simulink model "EKF_SIL_02"  (R2015a)
settings: Solver=ode45  StartTime=0.0  StopTime=totalSimulationTime  RelTol=1e-3
model workspace: external: MATLAB File Init_Model_02_Simulink.m (data not in the file)
undefined symbols (not defined in the file): Cov_nu, Cov_r, e_force_x, e_force_y, e_force_z, ieps, ita, lenLinks, n, P_d, P_k, p_x, p_y, p_z, parameter_gravitation, rho, rho_c, sig_f, sig_tau, t_delta, t_Kalman, tau_1, tau_2, tau_3, U_n_d, W_0, X_a_0, x_d, x_k
libraries: simulink x9, aerolibtransform2 x3, dspmtrx3 x2, visionstatistics x1, aerolibutil x1, visionsinks x1
(part 2 of 5)

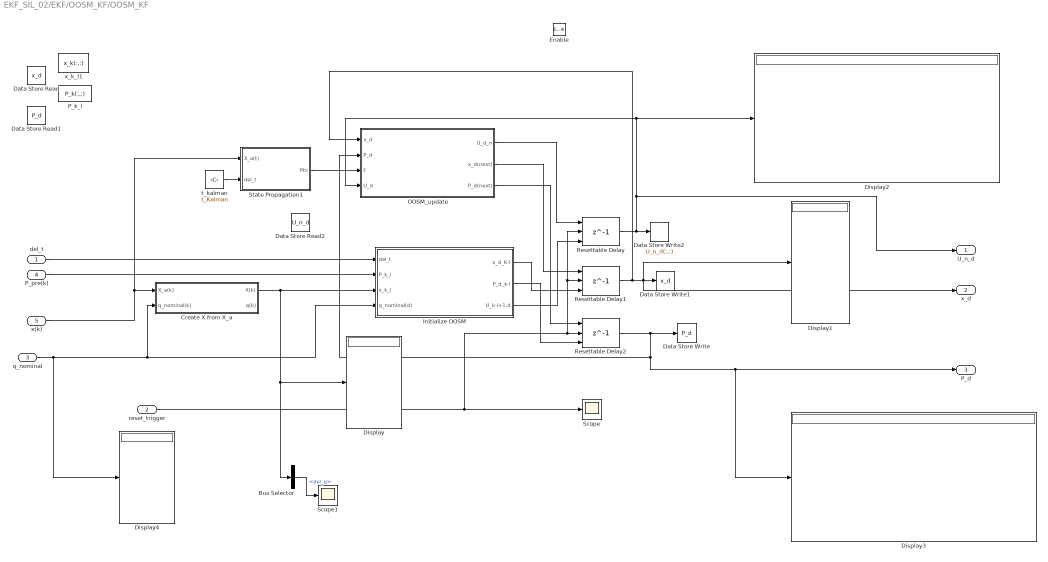
== system EKF_SIL_02/EKF/OOSM_KF/OOSM_KF ==
  del_t : Inport
  reset_trigger : Inport  Port=2
  q_nominal : Inport  Port=3
  P_pre(k) : Inport  Port=4
  "x(k) " : Inport  Port=5
  Enable : EnablePort
  Bus Selector : BusSelector  OutputSignals=del_q
  Create X from X_a : Subsystem
  Data Store Read : DataStoreRead  DataStoreName=x_d
  Data Store Read1 : DataStoreRead  DataStoreName=P_d
  Data Store Read2 : DataStoreRead  DataStoreName=U_n_d
  Data Store Write : DataStoreWrite  DataStoreName=P_d
  Data Store Write1 : DataStoreWrite  DataStoreName=x_d
  Data Store Write2 : DataStoreWrite  DataStoreName=U_n_d  DataStoreElements=U_n_d(:,:)
  Display{,1..4} (5 alike) : Display
  Initialize OOSM : Subsystem  TreatAsAtomicUnit=on
  OOSM_update : Subsystem
  P_k_l : DataStoreRead  DataStoreName=P_k  DataStoreElements=P_k(:,:)
  Resettable Delay : Delay  DelayLength=1  InitialConditionSource=Input port  ExternalReset=Rising
      settings: InputPortMap=u0,r5,p4
  Resettable Delay1 : Delay  DelayLength=1  InitialConditionSource=Input port  ExternalReset=Rising
      settings: InputPortMap=u0,r5,p4
  Resettable Delay2 : Delay  DelayLength=1  InitialConditionSource=Input port  ExternalReset=Rising
      settings: InputPortMap=u0,r5,p4
  Scope : Scope
      settings: SaveName=ScopeData10
  Scope1 : Scope
      settings: YMin=-0.8  YMax=0.4  SaveName=ScopeData17
  State Propagation1 : Subsystem
  t_kalman : Constant  Value=t_Kalman
  x_k_l1 : DataStoreRead  DataStoreName=x_k  DataStoreElements=x_k(:,:)
  U_n_d : Outport
  x_d : Outport  Port=2
  P_d : Outport  Port=3
  wires:
  del_t/1 -> Initialize OOSM/1(del_t)
  Initialize OOSM/3(U_k-l+1,d) -> Resettable Delay/3
  OOSM_update/1(U_d_n) -> Resettable Delay/1
  State Propagation1/1(Phi) -> OOSM_update/3(F)
  t_kalman/1 -> State Propagation1/2(del_t)
  Initialize OOSM/1(x_d_K-l) -> Resettable Delay1/3
  Resettable Delay1/1 -> OOSM_update/1(x_d), x_d/1, Display1/1, Data Store Write1/1
  Resettable Delay2/1 -> OOSM_update/2(P_d), Display3/1, P_d/1, Data Store Write/1
  reset_trigger/1 -> Resettable Delay/2, Resettable Delay1/2, Resettable Delay2/2, Scope/1
  Resettable Delay/1 -> Display2/1, OOSM_update/4("U_d "), U_n_d/1, Data Store Write2/1
  P_pre(k)/1 -> Initialize OOSM/2(P_k_l)
  q_nominal/1 -> Display4/1, Initialize OOSM/4(q_nominal(d)), Create X from X_a/2(q_nominal(k))
  OOSM_update/2(x_d(next)) -> Resettable Delay1/1
  OOSM_update/3(P_d(next)) -> Resettable Delay2/1
  Initialize OOSM/2(P_d_k-l) -> Resettable Delay2/3
  "x(k) "/1 -> State Propagation1/1("X_a(t)\t"), Create X from X_a/1(X_a(k))
  Create X from X_a/1(X(k)) -> Bus Selector/1, Display/1, Initialize OOSM/3(x_k_l)
  Bus Selector/1 -> Scope1/1  "<del_q>"

== system EKF_SIL_02/EKF/OOSM_KF/OOSM_enable ==
  "timestamp_cap " : Inport
  meas_packet : Inport  Port=2
  Bus Selector : BusSelector  OutputSignals=timestamp_processed
  Chart : Stateflow chart  TreatAsAtomicUnit=on
  Create nominal q(d) : Subsystem  TreatAsAtomicUnit=on
  Data Store Write : DataStoreWrite  DialogController=Simulink.DDGSource  DataStoreName=q_nominal_d
  Delay : Delay  DelayLength=1  InitialCondition=0
  Delay1 : Delay  DelayLength=1  InitialCondition=0
  Detect Increase : simulink/Logic and Bit Operations/Detect Increase  vinit=-1  InputProcessing=Inherited  OutDataTypeStr=boolean
  Detect Increase1 : simulink/Logic and Bit Operations/Detect Increase  vinit=-1  InputProcessing=Inherited  OutDataTypeStr=boolean
  Display : Display
  Enabled Subsystem : Subsystem  TreatAsAtomicUnit=on
  IC : InitialCondition  Value=-1
  IC1 : InitialCondition  Value=-1
  Mux : Mux  Inputs=2
  Scope : Scope
      settings: SaveName=ScopeData16
  Trigger : Outport
  reset_trigger : Outport  Port=2
  "q_nominal " : Outport  Port=3
  wires:
  Mux/1 -> Chart/Trigger
  Bus Selector/1 -> IC1/1  "<timestamp_processed>"
  meas_packet/1 -> Bus Selector/1
  IC1/1 -> Detect Increase1/1
  Detect Increase/1 -> Create nominal q(d)/Trigger, Delay/1  "camera_cap"
  Chart/1(out) -> Scope/1, Trigger/1
  "timestamp_cap "/1 -> IC/1
  IC/1 -> Create nominal q(d)/1(timestamp_cap), Detect Increase/1
  Detect Increase1/1 -> Delay1/1  "meas_arrived"
  Create nominal q(d)/1(q_nominal) -> Display/1, Data Store Write/1, "q_nominal "/1
  Delay/1 -> Mux/2, reset_trigger/1
  Delay1/1 -> Mux/1

== system EKF_SIL_02/EKF/Predictor/Create Bus [State Vector,X_a] ==
  X : Inport
  Bus Creator2 : BusCreator
  Bus Creator3 : BusCreator  Inputs=3
  Bus Creator4 : BusCreator  Inputs=3
  Bus Creator5 : BusCreator  Inputs=3
  Bus Creator6 : BusCreator
  Demux1 : Demux  Outputs=13
  X_bus : Outport
  wires:
  Bus Creator2/1 -> Bus Creator6/1  "q_est"
  Bus Creator3/1 -> Bus Creator6/2  "omega"
  Bus Creator4/1 -> Bus Creator6/3  "r"
  Bus Creator5/1 -> Bus Creator6/4  "r_dot"
  Bus Creator6/1 -> X_bus/1
  X/1 -> Demux1/1
  Demux1/1 -> Bus Creator2/1  "q_est_1"
  Demux1/2 -> Bus Creator2/2  "q_est_2"
  Demux1/3 -> Bus Creator2/3  "q_est_3"
  Demux1/4 -> Bus Creator2/4  "q_est_0"
  Demux1/5 -> Bus Creator3/1  "omega_x"
  Demux1/6 -> Bus Creator3/2  "omega_y"
  Demux1/7 -> Bus Creator3/3  "omega_z"
  Demux1/8 -> Bus Creator4/1  "r_x"
  Demux1/9 -> Bus Creator4/2  "r_y"
  Demux1/10 -> Bus Creator4/3  "r_z"
  Demux1/11 -> Bus Creator5/1  "r_x_dot"
  Demux1/12 -> Bus Creator5/2  "r_y_dot"
  Demux1/13 -> Bus Creator5/3  "r_z_dot"

== system EKF_SIL_02/EKF/Predictor/Create Bus [State Vector,X_a]1 ==
  X : Inport
  Bus Creator2 : BusCreator
  Bus Creator3 : BusCreator  Inputs=3
  Bus Creator4 : BusCreator  Inputs=3
  Bus Creator5 : BusCreator  Inputs=3
  Bus Creator6 : BusCreator
  Demux1 : Demux  Outputs=13
  X_bus : Outport
  wires:
  Demux1/13 -> Bus Creator5/3  "r_z_dot"
  Demux1/12 -> Bus Creator5/2  "r_y_dot"
  Demux1/11 -> Bus Creator5/1  "r_x_dot"
  Demux1/10 -> Bus Creator4/3  "r_z"
  Demux1/9 -> Bus Creator4/2  "r_y"
  Demux1/8 -> Bus Creator4/1  "r_x"
  Demux1/7 -> Bus Creator3/3  "omega_z"
  Demux1/6 -> Bus Creator3/2  "omega_y"
  Demux1/5 -> Bus Creator3/1  "omega_x"
  Demux1/4 -> Bus Creator2/4  "q_est_0"
  Demux1/3 -> Bus Creator2/3  "q_est_3"
  Demux1/2 -> Bus Creator2/2  "q_est_2"
  Demux1/1 -> Bus Creator2/1  "q_est_1"
  X/1 -> Demux1/1
  Bus Creator6/1 -> X_bus/1
  Bus Creator5/1 -> Bus Creator6/4  "r_dot"
  Bus Creator4/1 -> Bus Creator6/3  "r"
  Bus Creator3/1 -> Bus Creator6/2  "omega"
  Bus Creator2/1 -> Bus Creator6/1  "q_est"

== system EKF_SIL_02/EKF/Predictor/Create Bus [State Vector,X_a]2 ==
  X : Inport
  Bus Creator2 : BusCreator
  Bus Creator3 : BusCreator  Inputs=3
  Bus Creator4 : BusCreator  Inputs=3
  Bus Creator5 : BusCreator  Inputs=3
  Bus Creator6 : BusCreator
  Demux1 : Demux  Outputs=13
  X_bus : Outport
  wires:
  Demux1/13 -> Bus Creator5/3  "r_z_dot"
  Demux1/12 -> Bus Creator5/2  "r_y_dot"
  Demux1/11 -> Bus Creator5/1  "r_x_dot"
  Demux1/10 -> Bus Creator4/3  "r_z"
  Demux1/9 -> Bus Creator4/2  "r_y"
  Demux1/8 -> Bus Creator4/1  "r_x"
  Demux1/7 -> Bus Creator3/3  "omega_z"
  Demux1/6 -> Bus Creator3/2  "omega_y"
  Demux1/5 -> Bus Creator3/1  "omega_x"
  Demux1/4 -> Bus Creator2/4  "q_est_0"
  Demux1/3 -> Bus Creator2/3  "q_est_3"
  Demux1/2 -> Bus Creator2/2  "q_est_2"
  Demux1/1 -> Bus Creator2/1  "q_est_1"
  X/1 -> Demux1/1
  Bus Creator6/1 -> X_bus/1
  Bus Creator5/1 -> Bus Creator6/4  "r_dot"
  Bus Creator4/1 -> Bus Creator6/3  "r"
  Bus Creator3/1 -> Bus Creator6/2  "omega"
  Bus Creator2/1 -> Bus Creator6/1  "q_est"

== system EKF_SIL_02/EKF/Predictor/Create Bus [State Vector,X_a]3 ==
  X : Inport
  Bus Creator2 : BusCreator
  Bus Creator3 : BusCreator  Inputs=3
  Bus Creator4 : BusCreator  Inputs=3
  Bus Creator5 : BusCreator  Inputs=3
  Bus Creator6 : BusCreator
  Demux1 : Demux  Outputs=13
  X_bus : Outport
  wires:
  Bus Creator2/1 -> Bus Creator6/1  "q_est"
  Bus Creator3/1 -> Bus Creator6/2  "omega"
  Bus Creator4/1 -> Bus Creator6/3  "r"
  Bus Creator5/1 -> Bus Creator6/4  "r_dot"
  Bus Creator6/1 -> X_bus/1
  X/1 -> Demux1/1
  Demux1/1 -> Bus Creator2/1  "q_est_1"
  Demux1/2 -> Bus Creator2/2  "q_est_2"
  Demux1/3 -> Bus Creator2/3  "q_est_3"
  Demux1/4 -> Bus Creator2/4  "q_est_0"
  Demux1/5 -> Bus Creator3/1  "omega_x"
  Demux1/6 -> Bus Creator3/2  "omega_y"
  Demux1/7 -> Bus Creator3/3  "omega_z"
  Demux1/8 -> Bus Creator4/1  "r_x"
  Demux1/9 -> Bus Creator4/2  "r_y"
  Demux1/10 -> Bus Creator4/3  "r_z"
  Demux1/11 -> Bus Creator5/1  "r_x_dot"
  Demux1/12 -> Bus Creator5/2  "r_y_dot"
  Demux1/13 -> Bus Creator5/3  "r_z_dot"

== system EKF_SIL_02/EKF/Predictor/Create State error covariance (P) ==
  X_a : Inport
  P_previous : Inport  Port=2
  Add : Sum
  Math Function : Math  Operator=transpose  SaturateOnIntegerOverflow=on
  Matrix Concatenate : Concatenate  Mode=Multidimensional array  ConcatenateDimension=2
  Matrix Concatenate1 : Concatenate  Mode=Multidimensional array
  Matrix Concatenate2 : Concatenate  Mode=Multidimensional array  ConcatenateDimension=2
  Process noise covariance [rotational] : Subsystem
  Process noise covariance [translational] : Subsystem
  Product : Product  Inputs=3  Multiplication=Matrix(*)
  State Propagation : Subsystem
  zeros(6,6) : Constant  Value=zeros(6,6)
  P_current : Outport
  wires:
  Math Function/1 -> Product/3
  P_previous/1 -> Product/2
  Add/1 -> P_current/1
  X_a/1 -> State Propagation/1("X_a(t)\t")
  Product/1 -> Add/2
  Matrix Concatenate1/1 -> Add/1
  Matrix Concatenate2/1 -> Matrix Concatenate1/2
  Matrix Concatenate/1 -> Matrix Concatenate1/1
  Process noise covariance [translational]/1(Q_t) -> Matrix Concatenate2/2
  zeros(6,6)/1 -> Matrix Concatenate2/1, Matrix Concatenate/2
  Process noise covariance [rotational]/1(Q_r) -> Matrix Concatenate/1
  State Propagation/1(Phi) -> Math Function/1, Product/1, Process noise covariance [rotational]/1(Phi)

== system EKF_SIL_02/EKF/Predictor/Dynamic Model (Differential equations)1 ==
  X_a(t) : Inport
  Dynamic Model (Differential equations) : Subsystem
  X_a_dot : Outport
  wires:
  Dynamic Model (Differential equations)/1(X_a(t+1)) -> X_a_dot/1
  X_a(t)/1 -> Dynamic Model (Differential equations)/1(X_a(t))

== system EKF_SIL_02/EKF/Predictor/Dynamic Model (Differential equations)2 ==
  X_a(t) : Inport
  "theta " : Inport  Port=2
  d_theta : Inport  Port=3
  T_ee : Inport  Port=4
  Dynamic Model (Differential equations) : Subsystem
  X_a_dot : Outport
  wires:
  X_a(t)/1 -> Dynamic Model (Differential equations)/1(X_a(t))
  Dynamic Model (Differential equations)/1(X_a(t+1)) -> X_a_dot/1
  "theta "/1 -> Dynamic Model (Differential equations)/2("theta ")
  d_theta/1 -> Dynamic Model (Differential equations)/3(d_theta)
  T_ee/1 -> Dynamic Model (Differential equations)/4(T_ee)

== system EKF_SIL_02/Plant/Dynamic Model (Differential equations)/Orbital Dynamics  ==
  r : Inport
  Mu : Inport  Port=2
  n : Inport  Port=3
  "r_dot " : Inport  Port=4
  " " : Constant  Value=[0;0]
  Add : Sum
  Create Skew Symmetric : Subsystem
  Divide : Product  Inputs=*/
  Divide1 : Product  Inputs=*/
  Fcn : Fcn  Expr=u(1)^3
  Fcn1 : Fcn  Expr=u(1)^(1/3)
  Gain : Gain  Gain=-2
  Product : Product  Multiplication=Matrix(*)
  Product1 : Product  Multiplication=Matrix(*)
  Product2 : Product  Multiplication=Matrix(*)
  Product3 : Product
  Product4 : Product
  Product5 : Product
  Sum : Sum  Inputs=+--++
  Vector Concatenate1 : Concatenate
  "conc_re " : Constant  Value=[0;0]
  "e_force " : Constant  Value=[e_force_x;e_force_y;e_force_z]
  "norm " : Subsystem
  re : Concatenate
  "r_ddot " : Outport
  wires:
  " "/1 -> Vector Concatenate1/1
  Create Skew Symmetric/1(skew symmetric Matrix) -> Product/1, Product1/1, Product2/1
  Product1/1 -> Product2/2
  Mu/1 -> Product5/1, Divide/1
  Product/1 -> Gain/1
  "conc_re "/1 -> re/2
  re/1 -> Product4/1, Add/2
  Product5/1 -> Divide1/1
  "norm "/1("norm ") -> Fcn/1
  n/1 -> Product3/2, Vector Concatenate1/2, Product3/1
  Product3/1 -> Divide/2, Product4/2
  Vector Concatenate1/1 -> Create Skew Symmetric/1(vector)
  Add/1 -> "norm "/1(vector), Product5/2
  Gain/1 -> Sum/1
  Product2/1 -> Sum/2
  r/1 -> Product1/2, Add/1
  Product4/1 -> Sum/4
  "r_dot "/1 -> Product/2
  Divide1/1 -> Sum/3
  Fcn1/1 -> re/1
  Fcn/1 -> Divide1/2
  Divide/1 -> Fcn1/1
  "e_force "/1 -> Sum/5
  Sum/1 -> "r_ddot "/1

== system EKF_SIL_02/Plant/Dynamic Model (Differential equations)/Quaternion Kinematics ==
  q : Inport
  omega_rel : Inport  Port=2
  Constant2 : Constant  Value=0.5
  MATLAB Function : MATLAB Function  TreatAsAtomicUnit=on
  Product : Product  Multiplication=Matrix(*)
  Product1 : Product
  flag : Constant
  q_dot : Outport
  wires:
  MATLAB Function/1(CrossTensor) -> Product/1
  flag/1 -> MATLAB Function/2(flag)
  Constant2/1 -> Product1/2
  q/1 -> MATLAB Function/1(q)
  omega_rel/1 -> Product/2
  Product1/1 -> q_dot/1
  Product/1 -> Product1/1

== system EKF_SIL_02/Plant/Dynamic Model (Differential equations)/Rotational Dynamics ==
  omega : Inport
  p : Inport  Port=2
  Add : Sum
  Create  J : Subsystem
  Create Psi : Subsystem
  Product : Product  Multiplication=Matrix(*)
  tau : Constant  Value=[tau_1;tau_2;tau_3]
  omega_dot : Outport
  wires:
  omega/1 -> Create Psi/1("omega ")
  Create Psi/1(Psi) -> Add/1
  Add/1 -> omega_dot/1
  Product/1 -> Add/2
  p/1 -> Create Psi/2(p), Create  J/1(p)
  Create  J/1("J_k ") -> Product/1
  tau/1 -> Product/2

== system EKF_SIL_02/Plots and display/Create Measurements [Pose]1/Create Measurements [Orientation]  ==
  q : Inport
  "ita " : Inport  Port=2
  Bus Creator : BusCreator
  Demux : Demux
  MATLAB Function : MATLAB Function  TreatAsAtomicUnit=on
  Product : Product  Multiplication=Matrix(*)
  "flag " : Constant  Value=0
  Mu : Outport
  wires:
  Product/1 -> Demux/1
  q/1 -> Product/2
  Bus Creator/1 -> Mu/1  "Mu"
  "ita "/1 -> MATLAB Function/1(q)
  MATLAB Function/1(CrossTensor) -> Product/1
  "flag "/1 -> MATLAB Function/2(flag)
  Demux/1 -> Bus Creator/1
  Demux/2 -> Bus Creator/2
  Demux/3 -> Bus Creator/3
  Demux/4 -> Bus Creator/4

== system EKF_SIL_02/Plots and display/Create Measurements [Pose]1/Create Measurements [Position] ==
  r : Inport
  q : Inport  Port=2
  rho : Inport  Port=3
  "rho_c " : Inport  Port=4
  Add : Sum  Inputs=+++
  Bus Creator : BusCreator  Inputs=3
  "Create Rotation Matrix " : Subsystem
  Demux : Demux  Outputs=3
  Product : Product  Multiplication=Matrix(*)
  r_c : Outport
  wires:
  Add/1 -> Demux/1
  r/1 -> Add/2
  Bus Creator/1 -> r_c/1  "r_c"
  q/1 -> "Create Rotation Matrix "/1(q)
  "rho_c "/1 -> Add/1
  rho/1 -> Product/2
  "Create Rotation Matrix "/1(R) -> Product/1
  Product/1 -> Add/3
  Demux/1 -> Bus Creator/1  "r_c_x"
  Demux/2 -> Bus Creator/2  "r_c_y"
  Demux/3 -> Bus Creator/3  "r_c_z"

== system EKF_SIL_02/Plots and display/Create Measurements [Pose]2/Create Measurements [Orientation]  ==
  q : Inport
  "ita " : Inport  Port=2
  "ieps " : Inport  Port=3
  Bus Creator : BusCreator
  Demux : Demux
  MATLAB Function : MATLAB Function  TreatAsAtomicUnit=on
  MATLAB Function1 : MATLAB Function  TreatAsAtomicUnit=on
  Product : Product  Multiplication=Matrix(*)
  Product1 : Product  Multiplication=Matrix(*)
  "flag " : Constant  Value=0
  Mu : Outport
  wires:
  Demux/4 -> Bus Creator/4
  Demux/3 -> Bus Creator/3
  Demux/2 -> Bus Creator/2
  Demux/1 -> Bus Creator/1
  "flag "/1 -> MATLAB Function1/2(flag), MATLAB Function/2(flag)
  MATLAB Function/1(CrossTensor) -> Product/1
  "ita "/1 -> MATLAB Function/1(q)
  Bus Creator/1 -> Mu/1  "Mu"
  q/1 -> Product/2
  Product/1 -> MATLAB Function1/1(q)
  MATLAB Function1/1(CrossTensor) -> Product1/1
  "ieps "/1 -> Product1/2
  Product1/1 -> Demux/1

== system EKF_SIL_02/Plots and display/Create Measurements [Pose]2/Create Measurements [Position] ==
  r : Inport
  q : Inport  Port=2
  rho : Inport  Port=3
  "rho_c " : Inport  Port=4
  "ieps " : Inport  Port=5
  Add : Sum
  Add1 : Sum
  Bus Creator : BusCreator  Inputs=3
  "Create Rotation Matrix " : Subsystem
  Create Rotation Matrix 1 : Subsystem
  Demux : Demux  Outputs=3
  Product : Product  Multiplication=Matrix(*)
  Product1 : Product  Multiplication=Matrix(*)
  r_c : Outport
  wires:
  Demux/3 -> Bus Creator/3  "r_c_z"
  Demux/2 -> Bus Creator/2  "r_c_y"
  Demux/1 -> Bus Creator/1  "r_c_x"
  Product/1 -> Add/2
  "Create Rotation Matrix "/1(R) -> Product/1
  rho/1 -> Product/2
  q/1 -> "Create Rotation Matrix "/1(q)
  Bus Creator/1 -> r_c/1  "r_c"
  r/1 -> Add/1
  Create Rotation Matrix 1/1(R) -> Product1/1
  "rho_c "/1 -> Add1/2
  Add1/1 -> Demux/1
  Add/1 -> Product1/2
  "ieps "/1 -> Create Rotation Matrix 1/1(q)
  Product1/1 -> Add1/1

== system EKF_SIL_02/EKF/Measurement Update/Create X from X_a/Create Bus [State Vector,X_a]1 ==
  X : Inport
  Bus Creator2 : BusCreator
  Bus Creator3 : BusCreator  Inputs=3
  Bus Creator4 : BusCreator  Inputs=3
  Bus Creator5 : BusCreator  Inputs=3
  Bus Creator6 : BusCreator
  Demux1 : Demux  Outputs=13
  X_bus : Outport
  wires:
  Demux1/13 -> Bus Creator5/3  "r_z_dot"
  Demux1/12 -> Bus Creator5/2  "r_y_dot"
  Demux1/11 -> Bus Creator5/1  "r_x_dot"
  Demux1/10 -> Bus Creator4/3  "r_z"
  Demux1/9 -> Bus Creator4/2  "r_y"
  Demux1/8 -> Bus Creator4/1  "r_x"
  Demux1/7 -> Bus Creator3/3  "omega_z"
  Demux1/6 -> Bus Creator3/2  "omega_y"
  Demux1/5 -> Bus Creator3/1  "omega_x"
  Demux1/4 -> Bus Creator2/4  "q_est_0"
  Demux1/3 -> Bus Creator2/3  "q_est_3"
  Demux1/2 -> Bus Creator2/2  "q_est_2"
  Demux1/1 -> Bus Creator2/1  "q_est_1"
  X/1 -> Demux1/1
  Bus Creator6/1 -> X_bus/1
  Bus Creator5/1 -> Bus Creator6/4  "r_dot"
  Bus Creator4/1 -> Bus Creator6/3  "r"
  Bus Creator3/1 -> Bus Creator6/2  "omega"
  Bus Creator2/1 -> Bus Creator6/1  "q_est"

== system EKF_SIL_02/EKF/Measurement Update/Create X from X_a/Create Bus [State Vector] ==
  X : Inport
  Bus Creator{2..5} (4 alike) : BusCreator  Inputs=3
  Bus Creator6 : BusCreator
  Demux1 : Demux  Outputs=12
  X_bus : Outport
  wires:
  Demux1/4 -> Bus Creator3/1  "omega_x"
  Bus Creator2/1 -> Bus Creator6/1  "del_q"
  Demux1/8 -> Bus Creator4/2  "r_y"
  Demux1/6 -> Bus Creator3/3  "omega_z"
  Demux1/7 -> Bus Creator4/1  "r_x"
  Demux1/10 -> Bus Creator5/1  "r_x_dot"
  Bus Creator3/1 -> Bus Creator6/2  "omega"
  Demux1/3 -> Bus Creator2/3  "del_q_3"
  Demux1/1 -> Bus Creator2/1  "del_q_1"
  Demux1/11 -> Bus Creator5/2  "r_y_dot"
  Demux1/12 -> Bus Creator5/3  "r_z_dot"
  Demux1/2 -> Bus Creator2/2  "del_q_2"
  Demux1/5 -> Bus Creator3/2  "omega_y"
  Demux1/9 -> Bus Creator4/3  "r_z"
  Bus Creator4/1 -> Bus Creator6/3  "r"
  Bus Creator5/1 -> Bus Creator6/4  "r_dot"
  Bus Creator6/1 -> X_bus/1
  X/1 -> Demux1/1

== system EKF_SIL_02/EKF/Measurement Update/Create X from X_a/Create del_q [Intermediate stage] ==
  q : Inport
  q_nominal : Inport  Port=2
  Constant : Constant  Value=0
  Demux : Demux
  MATLAB Function : MATLAB Function  TreatAsAtomicUnit=on
  Mux : Mux  Inputs=3
  Product : Product  Multiplication=Matrix(*)
  Scope : Scope
      settings: SaveName=ScopeData6
  q_star : Subsystem
  del_q : Outport
  wires:
  q_star/1(q_star) -> Product/2
  MATLAB Function/1(CrossTensor) -> Product/1
  q/1 -> MATLAB Function/1(q)
  Constant/1 -> MATLAB Function/2(flag)
  q_nominal/1 -> q_star/1(q)
  Product/1 -> Demux/1
  Demux/1 -> Mux/1
  Demux/2 -> Mux/2
  Demux/3 -> Mux/3
  Mux/1 -> del_q/1
  Demux/4 -> Scope/1

== system EKF_SIL_02/EKF/Measurement Update/Update with K(d) and update current state/Create Bus [State Vector] ==
  X : Inport
  Bus Creator{2..5} (4 alike) : BusCreator  Inputs=3
  Bus Creator6 : BusCreator
  Demux1 : Demux  Outputs=12
  X_bus : Outport
  wires:
  Demux1/4 -> Bus Creator3/1  "omega_x"
  Bus Creator2/1 -> Bus Creator6/1  "del_q"
  Demux1/8 -> Bus Creator4/2  "r_y"
  Demux1/6 -> Bus Creator3/3  "omega_z"
  Demux1/7 -> Bus Creator4/1  "r_x"
  Demux1/10 -> Bus Creator5/1  "r_x_dot"
  Bus Creator3/1 -> Bus Creator6/2  "omega"
  Demux1/3 -> Bus Creator2/3  "del_q_3"
  Demux1/1 -> Bus Creator2/1  "del_q_1"
  Demux1/11 -> Bus Creator5/2  "r_y_dot"
  Demux1/12 -> Bus Creator5/3  "r_z_dot"
  Demux1/2 -> Bus Creator2/2  "del_q_2"
  Demux1/5 -> Bus Creator3/2  "omega_y"
  Demux1/9 -> Bus Creator4/3  "r_z"
  Bus Creator4/1 -> Bus Creator6/3  "r"
  Bus Creator5/1 -> Bus Creator6/4  "r_dot"
  Bus Creator6/1 -> X_bus/1
  X/1 -> Demux1/1

== system EKF_SIL_02/EKF/Measurement Update/Update with K(d) and update current state/Create H_k1 ==
  rho : Inport
  q_nominal : Inport  Port=2
  "Create Rotation Matrix " : Subsystem
  Create Skew Symmetric : Subsystem
  Gain : Gain  Gain=-2
  Matrix Concatenate : Concatenate  NumInputs=4  Mode=Multidimensional array  ConcatenateDimension=2
  Matrix Concatenate1 : Concatenate  NumInputs=4  Mode=Multidimensional array  ConcatenateDimension=2
  Matrix Concatenate2 : Concatenate  Mode=Multidimensional array
  Product : Product  Multiplication=Matrix(*)
  eye_3_3 : Constant  Value=eye(3,3)
  zeros_3_3 : Constant  Value=zeros(3,3)
  H_k : Outport
  wires:
  Matrix Concatenate/1 -> Matrix Concatenate2/1
  Matrix Concatenate1/1 -> Matrix Concatenate2/2
  rho/1 -> Create Skew Symmetric/1(vector)
  Gain/1 -> Matrix Concatenate/1
  Create Skew Symmetric/1(skew symmetric Matrix) -> Product/2
  zeros_3_3/1 -> Matrix Concatenate/2, Matrix Concatenate/4, Matrix Concatenate1/3, Matrix Concatenate1/4, Matrix Concatenate1/2
  eye_3_3/1 -> Matrix Concatenate/3, Matrix Concatenate1/1
  Product/1 -> Gain/1
  "Create Rotation Matrix "/1(R) -> Product/1
  Matrix Concatenate2/1 -> H_k/1
  q_nominal/1 -> "Create Rotation Matrix "/1(q)

== system EKF_SIL_02/EKF/Measurement Update/Update with K(d) and update current state/Create X_a from X1 ==
  q_nominal : Inport
  X : Inport  Port=2
  Bus Creator2 : BusCreator
  Bus Creator3 : BusCreator
  Bus Selector2 : BusSelector  OutputSignals=del_q
  Bus Selector3 : BusSelector  OutputSignals=omega,r,r_dot
  Create Bus [State Vector]1 : Subsystem
  "Create q_nominal " : Subsystem
  Demux : Demux
  Display1 : Display
  Display2 : Display
  Signal Conversion : SignalConversion
  X_a(k+1) : Outport
  X_a(internal) : Outport  Port=2
  "X(reduced) " : Outport  Port=3
  wires:
  Signal Conversion/1 -> X_a(k+1)/1
  "Create q_nominal "/1(q_est) -> Demux/1, Display1/1
  q_nominal/1 -> "Create q_nominal "/2(q_nominal)
  Bus Selector2/1 -> Display2/1, "Create q_nominal "/1(del_q)  "<del_q>"
  Bus Creator2/1 -> Signal Conversion/1, X_a(internal)/1
  Demux/3 -> Bus Creator3/3  "q_est_3"
  Demux/4 -> Bus Creator3/4  "q_est_0"
  Demux/2 -> Bus Creator3/2  "q_est_2"
  Bus Selector3/1 -> Bus Creator2/2  "<omega>"
  X/1 -> Create Bus [State Vector]1/1(X)
  Create Bus [State Vector]1/1(X_bus) -> Bus Selector2/1, Bus Selector3/1, "X(reduced) "/1
  Bus Creator3/1 -> Bus Creator2/1  "q_est"
  Bus Selector3/2 -> Bus Creator2/3  "<r>"
  Demux/1 -> Bus Creator3/1  "q_est_1"
  Bus Selector3/3 -> Bus Creator2/4  "<r_dot>"

== system EKF_SIL_02/EKF/Measurement Update/Update with K(d) and update current state/Create h_d ==
  rho : Inport
  del_q : Inport  Port=2
  q_nominal : Inport  Port=3
  r : Inport  Port=4
  Add : Sum
  "Create Rotation Matrix " : Subsystem
  Display : Display
  Product : Product  Multiplication=Matrix(*)
  Product1 : Product  Multiplication=Matrix(*)
  Subsystem : Subsystem
  Vector Concatenate1 : Concatenate
  h_d : Outport
  wires:
  Subsystem/1(h_1) -> Product/1
  Product/1 -> "Create Rotation Matrix "/1(q), Display/1
  Add/1 -> Vector Concatenate1/1
  Vector Concatenate1/1 -> h_d/1
  Product1/1 -> Add/1
  del_q/1 -> Vector Concatenate1/2, Subsystem/1(del_q)
  "Create Rotation Matrix "/1(R) -> Product1/1
  q_nominal/1 -> Product/2
  rho/1 -> Product1/2
  r/1 -> Add/2

== system EKF_SIL_02/EKF/Measurement Update/Update with K(d) and update current state/Create observation1 ==
  r_c : Inport
  Mu : Inport  Port=2
  rho_c : Inport  Port=3
  q_nominal : Inport  Port=4
  ita : Inport  Port=5
  0 : Constant  Value=0
  Add : Sum  Inputs=+-
  Bus Creator : BusCreator  Inputs=2
  Demux : Demux
  MATLAB Function : MATLAB Function  TreatAsAtomicUnit=on
  MATLAB Function2 : MATLAB Function  TreatAsAtomicUnit=on
  Mux : Mux  Inputs=3
  Product : Product  Multiplication=Matrix(*)
  Product1 : Product  Multiplication=Matrix(*)
  flag : Constant  Value=0
  q_star : Subsystem
  q_star1 : Subsystem
  z_d : Outport
  wires:
  Mux/1 -> Bus Creator/2
  Demux/3 -> Mux/3
  Demux/2 -> Mux/2
  Demux/1 -> Mux/1
  Product1/1 -> Demux/1
  Bus Creator/1 -> z_d/1
  Add/1 -> Bus Creator/1
  q_star/1(q_star) -> Product/2
  ita/1 -> q_star1/1(q)
  Product/1 -> Product1/2
  0/1 -> MATLAB Function/2(flag)
  q_nominal/1 -> q_star/1(q)
  q_star1/1(q_star) -> MATLAB Function2/1(q)
  MATLAB Function/1(CrossTensor) -> Product/1
  Mu/1 -> MATLAB Function/1(q)
  flag/1 -> MATLAB Function2/2(flag)
  rho_c/1 -> Add/2
  MATLAB Function2/1(CrossTensor) -> Product1/1
  r_c/1 -> Add/1

== system EKF_SIL_02/EKF/Measurement Update/Update with K(d) and update current state/Kalman gain (K_d) ==
  H_k : Inport
  P_pre(d) : Inport  Port=2
  S_k : Inport  Port=3
  U_n_d : Inport  Port=4
  Add : Sum
  Data Store Read : DataStoreRead  DataStoreName=U_n_d
  Display{,1..4} (5 alike) : Display
  Math Function : Math  Operator=transpose  SaturateOnIntegerOverflow=on
  Product : Product  Inputs=3  Multiplication=Matrix(*)
  Product1 : Product  Inputs=*/  Multiplication=Matrix(*)
  Product2 : Product  Multiplication=Matrix(*)
  Scope : Scope
      settings: SaveName=ScopeData19
  K : Outport
  S_d : Outport  Port=2
  wires:
  H_k/1 -> Math Function/1, Product/1
  Math Function/1 -> Product/3, Product2/2
  Product2/1 -> Product1/1
  S_k/1 -> Display4/1, Add/2
  Add/1 -> Display3/1, S_d/1, Product1/2
  Product/1 -> Add/1
  U_n_d/1 -> Display/1, Product2/1
  P_pre(d)/1 -> Display1/1, Product/2
  Product1/1 -> Display2/1, K/1
  ? -> Scope/1

== system EKF_SIL_02/EKF/Measurement Update/Update with K(k) and predict current state/Create Bus [State Vector,X_a]3 ==
  X : Inport
  Bus Creator2 : BusCreator
  Bus Creator3 : BusCreator  Inputs=3
  Bus Creator4 : BusCreator  Inputs=3
  Bus Creator5 : BusCreator  Inputs=3
  Bus Creator6 : BusCreator
  Demux1 : Demux  Outputs=13
  X_bus : Outport
  wires:
  Demux1/13 -> Bus Creator5/3  "r_z_dot"
  Demux1/12 -> Bus Creator5/2  "r_y_dot"
  Demux1/11 -> Bus Creator5/1  "r_x_dot"
  Demux1/10 -> Bus Creator4/3  "r_z"
  Demux1/9 -> Bus Creator4/2  "r_y"
  Demux1/8 -> Bus Creator4/1  "r_x"
  Demux1/7 -> Bus Creator3/3  "omega_z"
  Demux1/6 -> Bus Creator3/2  "omega_y"
  Demux1/5 -> Bus Creator3/1  "omega_x"
  Demux1/4 -> Bus Creator2/4  "q_est_0"
  Demux1/3 -> Bus Creator2/3  "q_est_3"
  Demux1/2 -> Bus Creator2/2  "q_est_2"
  Demux1/1 -> Bus Creator2/1  "q_est_1"
  X/1 -> Demux1/1
  Bus Creator6/1 -> X_bus/1
  Bus Creator5/1 -> Bus Creator6/4  "r_dot"
  Bus Creator4/1 -> Bus Creator6/3  "r"
  Bus Creator3/1 -> Bus Creator6/2  "omega"
  Bus Creator2/1 -> Bus Creator6/1  "q_est"

== system EKF_SIL_02/EKF/Measurement Update/Update with K(k) and predict current state/Create H_k ==
  rho : Inport
  q_nominal : Inport  Port=2
  "Create Rotation Matrix " : Subsystem
  Create Skew Symmetric : Subsystem
  Gain : Gain  Gain=-2
  Matrix Concatenate : Concatenate  NumInputs=4  Mode=Multidimensional array  ConcatenateDimension=2
  Matrix Concatenate1 : Concatenate  NumInputs=4  Mode=Multidimensional array  ConcatenateDimension=2
  Matrix Concatenate2 : Concatenate  Mode=Multidimensional array
  Product : Product  Multiplication=Matrix(*)
  eye_3_3 : Constant  Value=eye(3,3)
  zeros_3_3 : Constant  Value=zeros(3,3)
  H_k : Outport
  wires:
  q_nominal/1 -> "Create Rotation Matrix "/1(q)
  Matrix Concatenate2/1 -> H_k/1
  "Create Rotation Matrix "/1(R) -> Product/1
  Product/1 -> Gain/1
  eye_3_3/1 -> Matrix Concatenate1/1, Matrix Concatenate/3
  zeros_3_3/1 -> Matrix Concatenate1/2, Matrix Concatenate1/4, Matrix Concatenate1/3, Matrix Concatenate/4, Matrix Concatenate/2
  Create Skew Symmetric/1(skew symmetric Matrix) -> Product/2
  Gain/1 -> Matrix Concatenate/1
  rho/1 -> Create Skew Symmetric/1(vector)
  Matrix Concatenate1/1 -> Matrix Concatenate2/2
  Matrix Concatenate/1 -> Matrix Concatenate2/1

== system EKF_SIL_02/EKF/Measurement Update/Update with K(k) and predict current state/Create X_a from X ==
  q_nominal : Inport
  X : Inport  Port=2
  Bus Creator2 : BusCreator
  Bus Creator3 : BusCreator
  Bus Selector2 : BusSelector  OutputSignals=del_q
  Bus Selector3 : BusSelector  OutputSignals=omega,r,r_dot
  Create Bus [State Vector]1 : Subsystem
  "Create q_nominal " : Subsystem
  Demux : Demux
  Display1 : Display
  Signal Conversion : SignalConversion
  X_a(k+1) : Outport
  X_a(internal) : Outport  Port=2
  "X(reduced) " : Outport  Port=3
  wires:
  Bus Selector3/3 -> Bus Creator2/4  "<r_dot>"
  Demux/1 -> Bus Creator3/1  "q_est_1"
  Bus Selector3/2 -> Bus Creator2/3  "<r>"
  Bus Creator3/1 -> Bus Creator2/1  "q_est"
  Create Bus [State Vector]1/1(X_bus) -> "X(reduced) "/1, Bus Selector3/1, Bus Selector2/1
  X/1 -> Create Bus [State Vector]1/1(X)
  Bus Selector3/1 -> Bus Creator2/2  "<omega>"
  Demux/2 -> Bus Creator3/2  "q_est_2"
  Demux/4 -> Bus Creator3/4  "q_est_0"
  Demux/3 -> Bus Creator3/3  "q_est_3"
  Bus Creator2/1 -> X_a(internal)/1, Signal Conversion/1
  Bus Selector2/1 -> "Create q_nominal "/1(del_q)  "<del_q>"
  q_nominal/1 -> "Create q_nominal "/2(q_nominal)
  "Create q_nominal "/1(q_est) -> Display1/1, Demux/1
  Signal Conversion/1 -> X_a(k+1)/1

== system EKF_SIL_02/EKF/Measurement Update/Update with K(k) and predict current state/Create h ==
  rho : Inport
  del_q : Inport  Port=2
  q_nominal : Inport  Port=3
  r : Inport  Port=4
  Add : Sum
  "Create Rotation Matrix " : Subsystem
  Product : Product  Multiplication=Matrix(*)
  Product1 : Product  Multiplication=Matrix(*)
  Subsystem : Subsystem
  Vector Concatenate1 : Concatenate
  h_k : Outport
  wires:
  r/1 -> Add/2
  rho/1 -> Product1/2
  q_nominal/1 -> Product/2
  "Create Rotation Matrix "/1(R) -> Product1/1
  del_q/1 -> Subsystem/1(del_q), Vector Concatenate1/2
  Vector Concatenate1/1 -> h_k/1
  Product/1 -> "Create Rotation Matrix "/1(q)
  Subsystem/1(h_1) -> Product/1
  Product1/1 -> Add/1
  Add/1 -> Vector Concatenate1/1

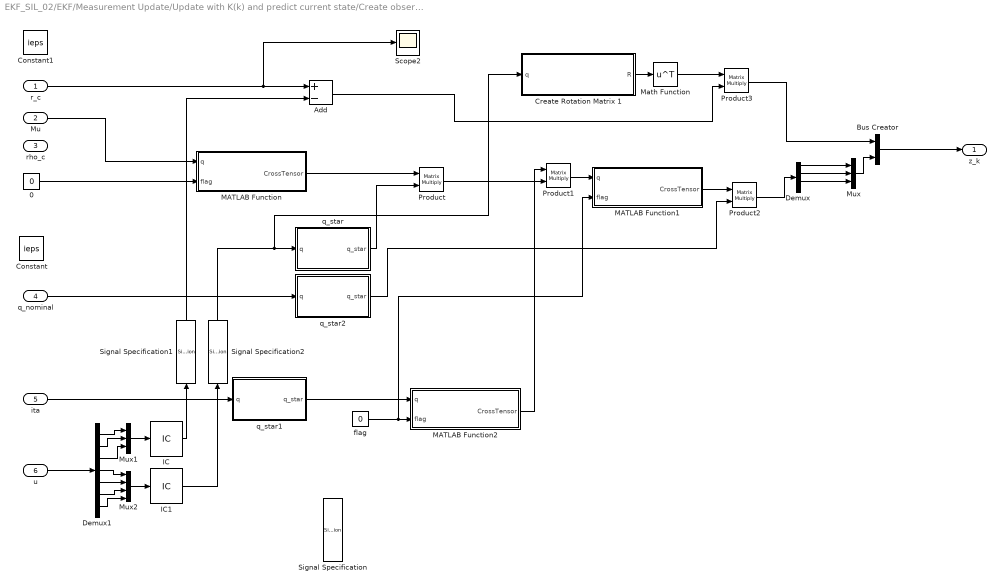
== system EKF_SIL_02/EKF/Measurement Update/Update with K(k) and predict current state/Create observation ==
  r_c : Inport
  Mu : Inport  Port=2
  rho_c : Inport  Port=3
  q_nominal : Inport  Port=4
  ita : Inport  Port=5
  u : Inport  Port=6
  0 : Constant  Value=0
  Add : Sum  Inputs=+-
  Bus Creator : BusCreator  Inputs=2
  Constant : Constant  Value=ieps
  Constant1 : Constant  Value=ieps
  Create Rotation Matrix 1 : Subsystem
  Demux : Demux
  Demux1 : Demux  Outputs=7
  IC : InitialCondition  Value=[-0.00036;-0.9865;-0.1854]
  IC1 : InitialCondition  Value=[-0.7071;0;0;0.7071]
  MATLAB Function : MATLAB Function  TreatAsAtomicUnit=on
  MATLAB Function1 : MATLAB Function  TreatAsAtomicUnit=on
  MATLAB Function2 : MATLAB Function  TreatAsAtomicUnit=on
  Math Function : Math  Operator=transpose  SaturateOnIntegerOverflow=on
  Mux : Mux  Inputs=3
  Mux1 : Mux  Inputs=3
  Mux2 : Mux
  Product{,1..3} (4 alike) : Product  Multiplication=Matrix(*)
  Scope2 : Scope
      settings: TimeRange=100  YMin=-0.2  YMax=1.6  SaveName=ScopeData30
  Signal Specification : SignalSpecification
  Signal Specification1 : SignalSpecification  Dimensions=[3,1]
  Signal Specification2 : SignalSpecification  Dimensions=[4,1]
  flag : Constant  Value=0
  q_star : Subsystem
  q_star1 : Subsystem
  q_star2 : Subsystem
  z_k : Outport
  wires:
  r_c/1 -> Scope2/1, Add/1
  MATLAB Function2/1(CrossTensor) -> Product1/1
  flag/1 -> MATLAB Function1/2(flag), MATLAB Function2/2(flag)
  Mu/1 -> MATLAB Function/1(q)
  MATLAB Function/1(CrossTensor) -> Product/1
  q_star1/1(q_star) -> MATLAB Function2/1(q)
  Product/1 -> Product1/2
  ita/1 -> q_star1/1(q)
  q_star/1(q_star) -> Product/2
  Bus Creator/1 -> z_k/1
  Product1/1 -> MATLAB Function1/1(q)
  Demux/1 -> Mux/1
  Demux/2 -> Mux/2
  Demux/3 -> Mux/3
  Mux/1 -> Bus Creator/2
  0/1 -> MATLAB Function/2(flag)
  Add/1 -> Product3/2
  Create Rotation Matrix 1/1(R) -> Math Function/1
  Math Function/1 -> Product3/1
  Product3/1 -> Bus Creator/1
  MATLAB Function1/1(CrossTensor) -> Product2/1
  Product2/1 -> Demux/1
  q_nominal/1 -> q_star2/1(q)
  q_star2/1(q_star) -> Product2/2
  u/1 -> Demux1/1
  Demux1/1 -> Mux1/1
  Demux1/2 -> Mux1/2
  Demux1/3 -> Mux1/3
  Demux1/4 -> Mux2/1
  Demux1/5 -> Mux2/2
  Demux1/6 -> Mux2/3
  Demux1/7 -> Mux2/4
  Mux2/1 -> IC1/1
  Mux1/1 -> IC/1
  IC/1 -> Signal Specification1/1
  IC1/1 -> Signal Specification2/1
  Signal Specification1/1 -> Add/2
  Signal Specification2/1 -> Create Rotation Matrix 1/1(q), q_star/1(q)

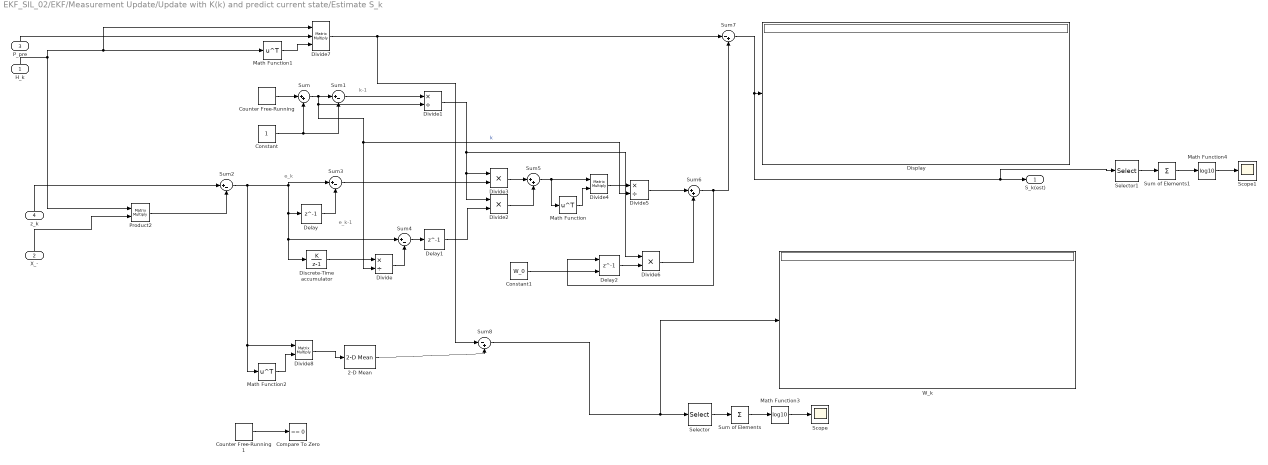
== system EKF_SIL_02/EKF/Measurement Update/Update with K(k) and predict current state/Estimate S_k ==
  note: k-1
  note: e_k-1
  note: e_k
  H_k : Inport
  X_- : Inport  Port=2
  P_pre : Inport  Port=3
  z_k : Inport  Port=4
  2-D Mean : visionstatistics/2-D Mean  run=on  reset_popup=None  directionMode=Entire input  dimension=1  treatSBRowAsCol=on  roiEnable=off  roiType=Rectangles  roiPortion=Entire ROI  roiOutput=Individual statistics for each ROI  roiFlag=off  outputDataTypeStr=Inherit: Same as accumulator  outputLastDataTypeStr=Inherit: Same as accumulator  outputMin=[]  outputMax=[]  accumMode=Binary point scaling  accumWordLength=32  accumFracLength=0  accumDataTypeStr=fixdt([],32,0)  accumLastDataTypeStr=fixdt([],32,0)  roundingMode=Floor  overflowMode=off
  Compare To Zero : simulink/Logic and Bit Operations/Compare To Zero  relop===  OutDataTypeStr=boolean
  Constant : Constant
  Constant1 : Constant  Value=W_0
  Counter Free-Running : simulink/Sources/Counter Free-Running  NumBits=16  tsamp=-1
  Counter Free-Running1 : simulink/Sources/Counter Free-Running  NumBits=10  tsamp=-1
  Delay : Delay  DelayLength=1  InitialCondition=0
  Delay1 : Delay  DelayLength=1  InitialCondition=0
  Delay2 : Delay  DelayLength=1  InitialConditionSource=Input port  InitialCondition=0
      settings: InputPortMap=u0,p4
  Discrete-Time accumulator : DiscreteIntegrator  IntegratorMethod=Accumulation: Forward Euler  InitialConditionSetting=State (most efficient)  SampleTime=-1
  Display : Display
  Divide : Product  Inputs=*/
  Divide1 : Product  Inputs=*/
  Divide2 : Product  Inputs=**
  Divide3 : Product  Inputs=**
  Divide4 : Product  Inputs=**  Multiplication=Matrix(*)
  Divide5 : Product  Inputs=*/
  Divide6 : Product  Inputs=**
  Divide7 : Product  Inputs=***  Multiplication=Matrix(*)
  Divide8 : Product  Inputs=**  Multiplication=Matrix(*)
  Math Function : Math  Operator=transpose  SaturateOnIntegerOverflow=on
  Math Function1 : Math  Operator=transpose  SaturateOnIntegerOverflow=on
  Math Function2 : Math  Operator=transpose  SaturateOnIntegerOverflow=on
  Math Function3 : Math  Operator=log10  SaturateOnIntegerOverflow=on
  Math Function4 : Math  Operator=log10  SaturateOnIntegerOverflow=on
  Product2 : Product  Multiplication=Matrix(*)
  Scope : Scope
      settings: YMin=-1.3  YMax=1  SaveName=ScopeData23
  Scope1 : Scope
      settings: YMin=-1.3  YMax=-0.1  SaveName=ScopeData26
  Selector : Selector  NumberOfDimensions=2  InputPortWidth=3  IndexOptions=Index vector (dialog),Index vector (dialog)  Indices=[1:6],[1:6]  OutputSizes=1,1
  Selector1 : Selector  NumberOfDimensions=2  InputPortWidth=3  IndexOptions=Index vector (dialog),Index vector (dialog)  Indices=[1:6],[1:6]  OutputSizes=1,1
  Sum : Sum  Inputs=|++
  Sum of Elements : Sum  Inputs=+
  Sum of Elements1 : Sum  Inputs=+
  Sum{1..4} (4 alike) : Sum  Inputs=|+-
  Sum5 : Sum  Inputs=|++
  Sum6 : Sum  Inputs=|++
  Sum7 : Sum  Inputs=|-+
  Sum8 : Sum  Inputs=|-+
  W_k : Display
  S_k(est) : Outport
  wires:
  Sum2/1 -> Math Function2/1, Divide8/1, Sum3/1, Sum4/1, Discrete-Time accumulator/1, Delay/1
  Constant1/1 -> Delay2/2
  Sum/1 -> Divide1/2, Divide5/2, Divide/2, Sum1/1  "k"
  Math Function/1 -> Divide4/2
  Delay2/1 -> Divide6/2
  Divide2/1 -> Sum5/2
  Discrete-Time accumulator/1 -> Divide/1
  Delay/1 -> Sum3/2
  Divide4/1 -> Divide5/1
  Sum4/1 -> Delay1/1
  Divide6/1 -> Sum6/2
  Divide/1 -> Sum4/2
  Math Function1/1 -> Divide7/3
  Sum5/1 -> Math Function/1, Divide4/1
  Divide1/1 -> Divide6/1, Divide3/1, Divide2/1
  Sum3/1 -> Divide3/2
  Divide3/1 -> Sum5/1
  Sum1/1 -> Divide1/1
  Delay1/1 -> Divide2/2
  Divide5/1 -> Sum6/1
  H_k/1 -> Product2/1, Math Function1/1, Divide7/1
  X_-/1 -> Product2/2
  z_k/1 -> Sum2/1
  P_pre/1 -> Divide7/2
  Constant/1 -> Sum1/2, Sum/2
  Counter Free-Running/1 -> Sum/1
  Divide7/1 -> Sum8/1, Sum7/1
  Sum6/1 -> Sum7/2, Delay2/1
  Product2/1 -> Sum2/2
  Math Function2/1 -> Divide8/2
  Divide8/1 -> 2-D Mean/1
  Counter Free-Running1/1 -> Compare To Zero/1
  2-D Mean/1 -> Sum8/2
  Selector/1 -> Sum of Elements/1
  Sum of Elements/1 -> Math Function3/1
  Math Function3/1 -> Scope/1
  Sum7/1 -> Selector1/1, S_k(est)/1, Display/1
  Selector1/1 -> Sum of Elements1/1
  Sum of Elements1/1 -> Math Function4/1
  Math Function4/1 -> Scope1/1
  Sum8/1 -> W_k/1, Selector/1

== system EKF_SIL_02/EKF/Measurement Update/Update with K(k) and predict current state/Kalman gain ==
  H_k : Inport
  P_pre : Inport  Port=2
  S_k : Inport  Port=3
  Add : Sum
  Math Function : Math  Operator=transpose  SaturateOnIntegerOverflow=on
  Math Function1 : Math  Operator=log10  SaturateOnIntegerOverflow=on
  Product : Product  Inputs=3  Multiplication=Matrix(*)
  Product1 : Product  Inputs=*/  Multiplication=Matrix(*)
  Product2 : Product  Multiplication=Matrix(*)
  Scope : Scope
      settings: YMin=-1.61  YMax=-1.41  SaveName=ScopeData22
  Selector : Selector  NumberOfDimensions=2  InputPortWidth=3  IndexOptions=Index vector (dialog),Index vector (dialog)  Indices=[1:6],[1:6]  OutputSizes=1,1
  Sum of Elements : Sum  Inputs=+
  K : Outport
  H.P(k|k-1).H' + S_k : Outport  Port=2
  H.P(k|k-1).H' : Outport  Port=3
  wires:
  Product/1 -> H.P(k|k-1).H'/1, Add/1
  Product2/1 -> Product1/1
  Math Function/1 -> Product2/2, Product/3
  H_k/1 -> Product/1, Math Function/1
  P_pre/1 -> Product2/1, Product/2
  Product1/1 -> K/1
  S_k/1 -> Add/2
  Add/1 -> H.P(k|k-1).H' + S_k/1, Selector/1, Product1/2
  Selector/1 -> Sum of Elements/1
  Sum of Elements/1 -> Math Function1/1
  Math Function1/1 -> Scope/1

== system EKF_SIL_02/EKF/Measurement Update/Update with K(k) and predict current state/Outlier rejector ==
  Computed K : Inport
  X^2 : Inport  Port=2
  Chi_threshold : Constant  Value=1000
  Relational Operator : RelationalOperator  Operator=<  OutDataTypeStr=boolean
  Scope : Scope
      settings: ShowLegends=on  SaveName=ScopeData31
  Switch : Switch  Criteria=u2 > Threshold
  zeros(12,) : Constant  Value=zeros(12,6)
  K (outlier_checked) : Outport
  wires:
  Computed K/1 -> Switch/1
  X^2/1 -> Relational Operator/1
  Chi_threshold/1 -> Relational Operator/2
  Relational Operator/1 -> Switch/2, Scope/1  "Outlier rejector (Not)"
  Switch/1 -> K (outlier_checked)/1
  zeros(12,)/1 -> Switch/3

== system EKF_SIL_02/EKF/Measurement Update/Update with K(k) and predict current state/Propagate_state (full) ==
  X_a(k-n) : Inport
  del_t : Inport  Port=2
  Bus Selector : BusSelector  OutputSignals=omega,r,r_dot
  Create q_nominal : Subsystem  TreatAsAtomicUnit=on
  Mux : Mux  Inputs=3
  Mux1 : Mux  Inputs=2
  Product : Product  Multiplication=Matrix(*)
  Selector : Selector  NumberOfDimensions=2  InputPortWidth=3  IndexOptions=Index vector (dialog),Index vector (dialog)  Indices=[4:12],[4:12]  OutputSizes=1,1
  State Propagation1 : Subsystem
  X_a(k) : Outport
  wires:
  X_a(k-n)/1 -> Bus Selector/1, Create q_nominal/1(X_a), State Propagation1/1("X_a(t)\t")
  Mux1/1 -> X_a(k)/1
  Bus Selector/1 -> Mux/1  "<omega>"
  Bus Selector/2 -> Mux/2  "<r>"
  Selector/1 -> Product/1
  Mux/1 -> Product/2
  Bus Selector/3 -> Mux/3  "<r_dot>"
  Product/1 -> Mux1/2
  Create q_nominal/1(Out1) -> Mux1/1
  State Propagation1/1(Phi) -> Selector/1
  del_t/1 -> Create q_nominal/2(del_t), State Propagation1/2(del_t)

== system EKF_SIL_02/EKF/OOSM_KF/OOSM_KF/Create X from X_a ==
  X_a(k) : Inport
  q_nominal(k) : Inport  Port=2
  Bus Creator1 : BusCreator
  Bus Selector3 : BusSelector  OutputSignals=q_est,omega,r,r_dot
  Bus Selector5 : BusSelector  OutputSignals=q_est
  Create Bus [State Vector,X_a]1 : Subsystem
  Create Bus [State Vector] : Subsystem
  Create del_q [Intermediate stage] : Subsystem
  IC : InitialCondition  Value=[X_a_0]
  X(k) : Outport
  q(k) : Outport  Port=2
  wires:
  Create Bus [State Vector,X_a]1/1(X_bus) -> Bus Selector3/1, Bus Selector5/1
  Create del_q [Intermediate stage]/1(del_q) -> Bus Creator1/1  "del_q"
  Bus Selector3/2 -> Bus Creator1/2  "<omega>"
  Bus Selector3/3 -> Bus Creator1/3  "<r>"
  Bus Selector3/4 -> Bus Creator1/4  "<r_dot>"
  Bus Creator1/1 -> Create Bus [State Vector]/1(X)
  Bus Selector5/1 -> Create del_q [Intermediate stage]/1(q)  "<q_est>"
  Create Bus [State Vector]/1(X_bus) -> X(k)/1
  X_a(k)/1 -> IC/1
  IC/1 -> Create Bus [State Vector,X_a]1/1(X)
  Bus Selector3/1 -> q(k)/1  "<q_est>"
  q_nominal(k)/1 -> Create del_q [Intermediate stage]/2(q_nominal)

== system EKF_SIL_02/EKF/OOSM_KF/OOSM_KF/Initialize OOSM ==
  del_t : Inport
  P_k_l : Inport  Port=2
  x_k_l : Inport  Port=3
  q_nominal(d) : Inport  Port=4
  Counter Free-Running : simulink/Sources/Counter Free-Running  NumBits=16  tsamp=-1
  Create Bus [State Vector] : Subsystem
  Create State error covariance (P) : Subsystem
  Data Store Write : DataStoreWrite  DataStoreName=flag_OOSM_update  DataStoreElements=flag_OOSM_update
  Display : Display
  Display3 : Display
  Display4 : Display
  Product2 : Product  Multiplication=Matrix(*)
  Propagate_state (full) : Subsystem
  Scope1 : Scope
      settings: SaveName=ScopeData2
  State Propagation : Subsystem
  Sum : Sum  Inputs=|+-
  t_Kalman : Constant  Value=t_Kalman
  true_flag : Constant  Value=true
  x_d_K-l : Outport
  P_d_k-l : Outport  Port=2
  U_k-l+1,d : Outport  Port=3
  wires:
  Product2/1 -> U_k-l+1,d/1
  del_t/1 -> Sum/2, Display4/1, Propagate_state (full)/2(del_t), Create State error covariance (P)/3(del_t)
  t_Kalman/1 -> Sum/1
  true_flag/1 -> Data Store Write/1
  Counter Free-Running/1 -> Scope1/1
  Sum/1 -> State Propagation/2(del_t), Display3/1
  P_k_l/1 -> Create State error covariance (P)/2(P_previous)
  Create State error covariance (P)/1(P_current) -> Product2/2, P_d_k-l/1
  Propagate_state (full)/1(X_a(k-n,d)) -> Create Bus [State Vector]/1(X), x_d_K-l/1
  State Propagation/1(Phi) -> Product2/1
  x_k_l/1 -> Propagate_state (full)/1(X_a(k-n)), Create State error covariance (P)/1(X_a)
  Create Bus [State Vector]/1(X_bus) -> State Propagation/1("X_a(t)\t")
  q_nominal(d)/1 -> Propagate_state (full)/3(q_nominal(d))

== system EKF_SIL_02/EKF/OOSM_KF/OOSM_KF/OOSM_update ==
  x_d : Inport
  P_d : Inport  Port=2
  F : Inport  Port=3
  "U_d " : Inport  Port=4
  Counter Free-Running : simulink/Sources/Counter Free-Running  NumBits=16  tsamp=-1
  Data Store Read : DataStoreRead  DataStoreName=U_n_d
  Data Store Write : DataStoreWrite  DialogController=Simulink.DDGSource  DataStoreName=x_d  DataStoreElements=x_d(:,:)
  Data Store Write1 : DataStoreWrite  DataStoreName=P_d  DataStoreElements=P_d(:,:)
  Data Store Write2 : DataStoreWrite  DataStoreName=U_n_d  DataStoreElements=U_n_d(:,:)
  Display1 : Display
  Display2 : Display
  Display3 : Display
  Product : Product  Multiplication=Matrix(*)
  Scope1 : Scope
      settings: SaveName=ScopeData13
  U_d_n : Outport
  x_d(next) : Outport  Port=2
  P_d(next) : Outport  Port=3
  wires:
  x_d/1 -> Display1/1, x_d(next)/1, Data Store Write/1
  P_d/1 -> Display2/1, P_d(next)/1, Data Store Write1/1
  F/1 -> Product/1
  "U_d "/1 -> Product/2
  Counter Free-Running/1 -> Scope1/1
  Product/1 -> Display3/1, U_d_n/1, Data Store Write2/1

== system EKF_SIL_02/EKF/OOSM_KF/OOSM_KF/State Propagation1 ==
  "X_a(t)\t" : Inport
  del_t : Inport  Port=2
  Create Bus [State Vector,X_a]2 : Subsystem
  Create M : Subsystem
  MATLAB Function : MATLAB Function  TreatAsAtomicUnit=on
  n : Constant  Value=n
  p : Constant  Value=[p_x;p_y;p_z]
  Phi : Outport
  wires:
  p/1 -> Create M/2(p), MATLAB Function/4(p)
  n/1 -> MATLAB Function/2(n)
  del_t/1 -> MATLAB Function/3(t_Kalman)
  MATLAB Function/1(Phi) -> Phi/1
  "X_a(t)\t"/1 -> Create Bus [State Vector,X_a]2/1(X), MATLAB Function/1(X_a)
  Create M/1(M) -> MATLAB Function/5(M)
  Create Bus [State Vector,X_a]2/1(X_bus) -> Create M/1("X_a ")

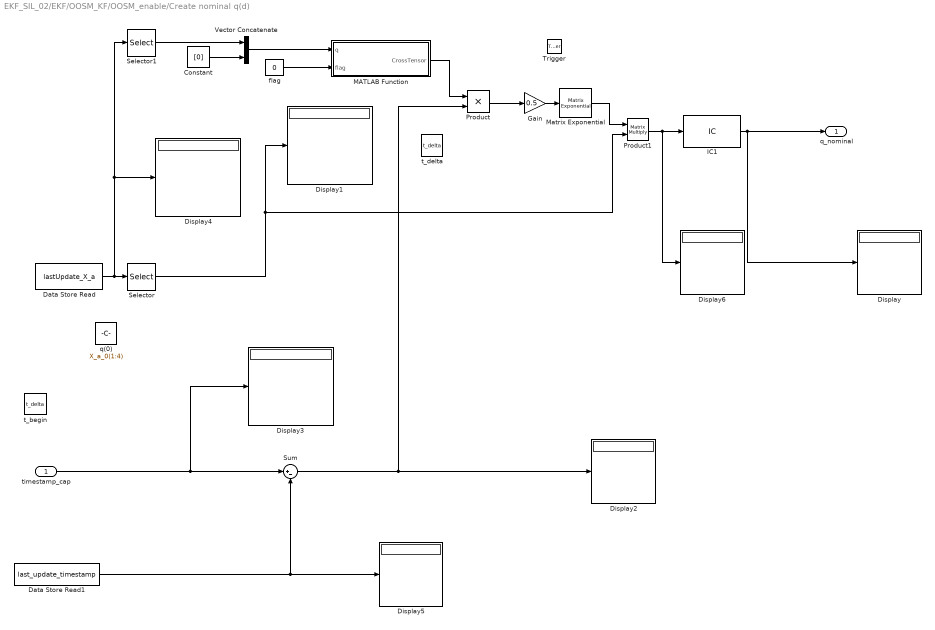
== system EKF_SIL_02/EKF/OOSM_KF/OOSM_enable/Create nominal q(d) ==
  timestamp_cap : Inport
  Trigger : TriggerPort  PortDimensions=1
  Constant : Constant  Value=[0]
  Data Store Read : DataStoreRead  DialogController=Simulink.DDGSource  DataStoreName=lastUpdate_X_a  DataStoreElements=lastUpdate_X_a
  Data Store Read1 : DataStoreRead  DataStoreName=last_update_timestamp
  Display{,1..6} (7 alike) : Display
  Gain : Gain  Gain=0.5
  IC1 : InitialCondition  Value=X_a_0(1:4)
  MATLAB Function : MATLAB Function  TreatAsAtomicUnit=on
  Matrix Exponential : dspmtrx3/Matrix Exponential
  Product : Product
  Product1 : Product  Multiplication=Matrix(*)
  Selector : Selector  InputPortWidth=13  Indices=[1:4]
  Selector1 : Selector  InputPortWidth=13  Indices=[5:7]
  Sum : Sum  Inputs=|+-
  Vector Concatenate : Concatenate
  flag : Constant  Value=0
  q(0) : Constant  Value=X_a_0(1:4)
  t_begin : Constant  Value=t_delta
  "t_delta " : Constant  Value=t_delta
  q_nominal : Outport
  wires:
  MATLAB Function/1(CrossTensor) -> Product/1
  Sum/1 -> Display2/1, Product/2
  Selector1/1 -> Vector Concatenate/1
  Constant/1 -> Vector Concatenate/2
  flag/1 -> MATLAB Function/2(flag)
  Product/1 -> Gain/1
  Vector Concatenate/1 -> MATLAB Function/1(q)
  Gain/1 -> Matrix Exponential/1
  Matrix Exponential/1 -> Product1/1
  IC1/1 -> Display/1, q_nominal/1
  Selector/1 -> Product1/2, Display1/1
  Data Store Read/1 -> Display4/1, Selector1/1, Selector/1
  timestamp_cap/1 -> Display3/1, Sum/1
  Data Store Read1/1 -> Sum/2, Display5/1
  Product1/1 -> Display6/1, IC1/1

== system EKF_SIL_02/EKF/OOSM_KF/OOSM_enable/Enabled Subsystem ==
  Enable : EnablePort
  Create H_k : Subsystem
  Data Store Read : DataStoreRead  DataStoreName=q_nominal_d
  "rho " : Constant  Value=rho
  wires:
  "rho "/1 -> Create H_k/1(rho)
  Data Store Read/1 -> Create H_k/2(q_nominal)

== system EKF_SIL_02/EKF/Predictor/Create State error covariance (P)/Process noise covariance [rotational] ==
  Phi : Inport
  Process Noise covariance : MATLAB Function  TreatAsAtomicUnit=on
  p : Constant  Value=[p_x;p_y;p_z]
  sig_tau : Constant  Value=sig_tau
  t_delta : Constant  Value=t_Kalman
  Q_r : Outport
  wires:
  Phi/1 -> Process Noise covariance/1(Phi)
  t_delta/1 -> Process Noise covariance/3(t_delta)
  sig_tau/1 -> Process Noise covariance/4(tau)
  p/1 -> Process Noise covariance/6(p)
  Process Noise covariance/1(Q_r) -> Q_r/1

== system EKF_SIL_02/EKF/Predictor/Create State error covariance (P)/Process noise covariance [translational] ==
  Process noise covariance [translational] : MATLAB Function  TreatAsAtomicUnit=on
  n : Constant  Value=n
  sig_f : Constant  Value=sig_f
  t_Kalman : Constant  Value=t_Kalman
  Q_t : Outport
  wires:
  n/1 -> Process noise covariance [translational]/2(n)
  t_Kalman/1 -> Process noise covariance [translational]/1(t_Kalman)
  sig_f/1 -> Process noise covariance [translational]/3(sigma_f)
  Process noise covariance [translational]/1(Q_t_k) -> Q_t/1

== system EKF_SIL_02/EKF/Predictor/Create State error covariance (P)/State Propagation ==
  "X_a(t)\t" : Inport
  Create M : Subsystem
  MATLAB Function : MATLAB Function  TreatAsAtomicUnit=on
  n : Constant  Value=n
  p : Constant  Value=[p_x;p_y;p_z]
  "t_Kalman " : Constant  Value=t_Kalman
  Phi : Outport
  wires:
  p/1 -> Create M/2(p), MATLAB Function/4(p)
  n/1 -> MATLAB Function/2(n)
  "t_Kalman "/1 -> MATLAB Function/3(t_Kalman)
  MATLAB Function/1(Phi) -> Phi/1
  "X_a(t)\t"/1 -> Create M/1("X_a "), MATLAB Function/1(X_a)
  Create M/1(M) -> MATLAB Function/5(M)

== system EKF_SIL_02/EKF/Predictor/Dynamic Model (Differential equations)1/Dynamic Model (Differential equations) ==
  X_a(t) : Inport
  Bus Creator : BusCreator
  Constant : Constant  Value=[0]  SampleTime=-1
  Constant1 : Constant  Value=zeros(3,1)  SampleTime=-1
  "Orbital Dynamics " : Subsystem
  Quaternion Kinematics : Subsystem
  Rotational Dynamics : Subsystem
  Vector Concatenate : Concatenate
  n : Constant  Value=n  SampleTime=-1
  omega : Selector  InputPortWidth=13  Indices=[5 6 7]
  p : Constant  Value=[p_x;p_y;p_z]  SampleTime=-1
  parameter_gravitation : Constant  Value=parameter_gravitation  SampleTime=-1
  q : Selector  InputPortWidth=13  Indices=[1 2 3 4]
  r : Selector  InputPortWidth=13  Indices=[8 9 10]
  r_dot : Selector  InputPortWidth=13  Indices=[11 12 13]
  X_a(t+1) : Outport
  wires:
  Constant/1 -> Vector Concatenate/2
  p/1 -> Rotational Dynamics/2(p)
  Vector Concatenate/1 -> Quaternion Kinematics/2(omega_rel)
  parameter_gravitation/1 -> "Orbital Dynamics "/2(Mu)
  n/1 -> "Orbital Dynamics "/3(n)
  Constant1/1 -> Bus Creator/4  "r_ddot"
  Quaternion Kinematics/1(q_dot) -> Bus Creator/1  "q_dot"
  Rotational Dynamics/1(omega_dot) -> Bus Creator/2  "omega_dot"
  X_a(t)/1 -> q/1, omega/1, r_dot/1, r/1
  q/1 -> Quaternion Kinematics/1(q)
  omega/1 -> Rotational Dynamics/1(omega), Vector Concatenate/1
  r/1 -> "Orbital Dynamics "/1(r)
  r_dot/1 -> "Orbital Dynamics "/4("r_dot "), Bus Creator/3
  Bus Creator/1 -> X_a(t+1)/1
